simulink model "AirDragTorque"  (R2024b)
settings: Solver=ode8  StartTime=0.0  StopTime=1000  FixedStep=0.1  RelTol=1e-3
undefined symbols (not defined in the file or in its folder): Earth, env, IC, orb, sat
libraries: matrix_library x14
settings Model: Creator=eleon  LastModifiedBy=eleon

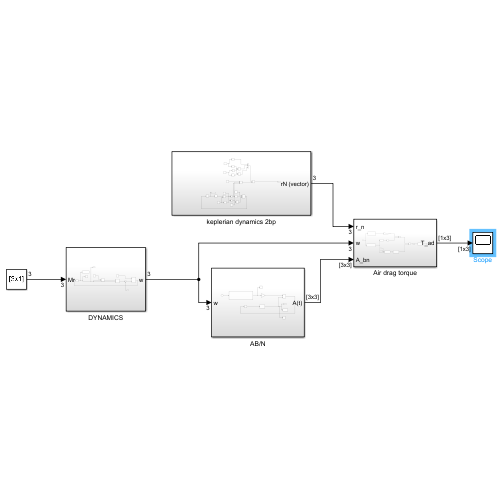
[thumbnail: Simulink's stored preview of the top-level diagram]
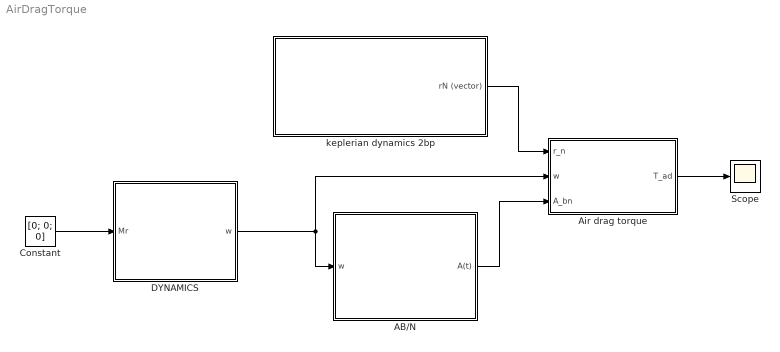
== system AirDragTorque ==
  AB/N : Subsystem
  Air drag torque : Subsystem
  Constant : Constant  Value=[0; 0; 0]
  DYNAMICS : Subsystem
  Scope : Scope
  keplerian dynamics 2bp : Subsystem
  wires:
  Air drag torque/1(T_ad) -> Scope/1
  DYNAMICS/1(w) -> AB/N/1(w), Air drag torque/2(w)
  AB/N/1(A(t)) -> Air drag torque/3(A_bn)
  Constant/1 -> DYNAMICS/1(Mr)
  keplerian dynamics 2bp/1(rN (vector)) -> Air drag torque/1(r_n)

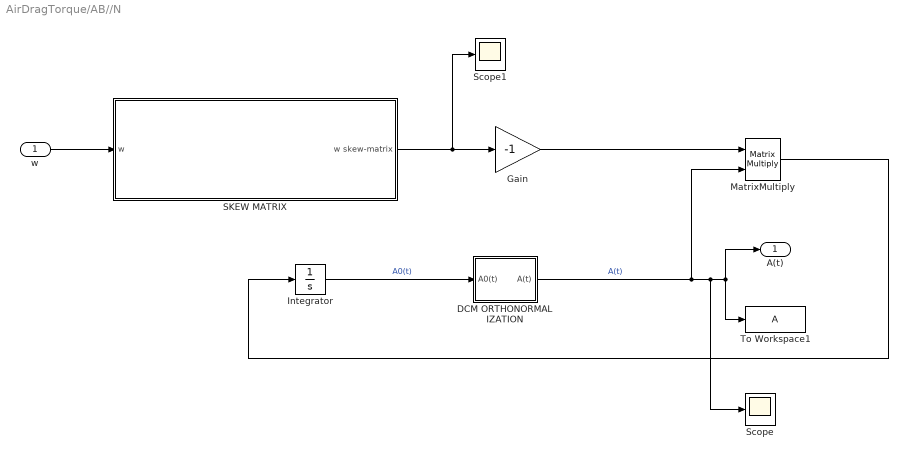
== system AirDragTorque/AB//N ==
  w : Inport
  DCM ORTHONORMALIZATION : Subsystem
  Gain : Gain  Gain=-1
  Integrator : Integrator  InitialCondition=eye(3)
  MatrixMultiply : Product  Multiplication=Matrix(*)
  SKEW MATRIX : Subsystem
  Scope : Scope
  Scope1 : Scope
  To Workspace1 : ToWorkspace  VariableName=A  SampleTime=-1
  A(t) : Outport
  wires:
  w/1 -> SKEW MATRIX/1(w)
  Gain/1 -> MatrixMultiply/1
  MatrixMultiply/1 -> Integrator/1
  SKEW MATRIX/1(w skew-matrix) -> Scope1/1, Gain/1
  Integrator/1 -> DCM ORTHONORMALIZATION/1(A0(t))  "A0(t)"
  DCM ORTHONORMALIZATION/1(A(t)) -> Scope/1, A(t)/1, To Workspace1/1, MatrixMultiply/2  "A(t)"

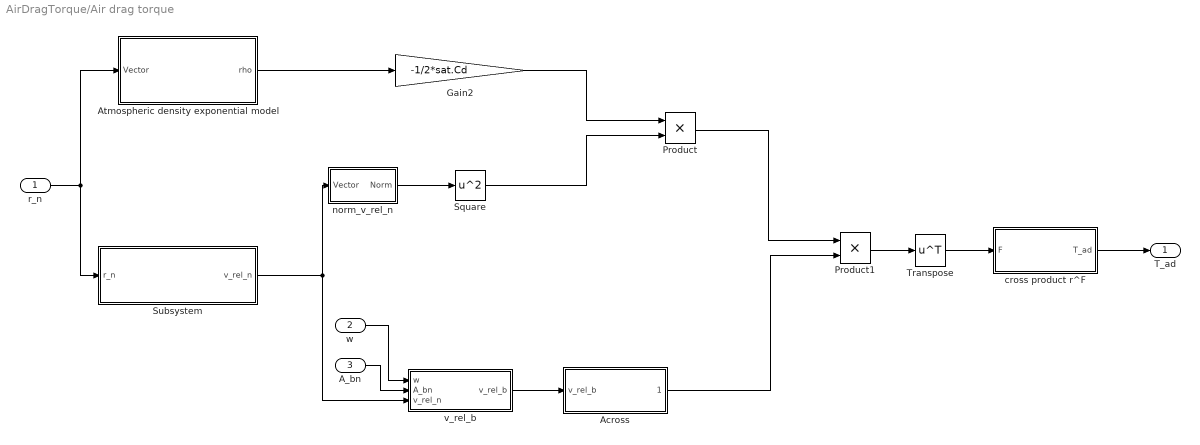
== system AirDragTorque/Air drag torque ==
  r_n : Inport
  w : Inport  Port=2
  A_bn : Inport  Port=3
  Across : Subsystem
  Atmospheric density exponential model : Subsystem
  Gain2 : Gain  Gain=-1/2*sat.Cd
  Product : Product
  Product1 : Product
  Square : Math  Operator=square
  Subsystem : Subsystem
  Transpose : Math  Operator=transpose
  cross product r^F : Subsystem
  norm_v_rel_n : Subsystem
  v_rel_b : Subsystem
  T_ad : Outport
  wires:
  r_n/1 -> Subsystem/1(r_n), Atmospheric density exponential model/1(Vector)
  Atmospheric density exponential model/1(rho) -> Gain2/1
  norm_v_rel_n/1(Norm) -> Square/1
  w/1 -> v_rel_b/1(w)
  A_bn/1 -> v_rel_b/2(A_bn)
  v_rel_b/1(v_rel_b) -> Across/1(v_rel_b)
  cross product r^F/1(T_ad) -> T_ad/1
  Gain2/1 -> Product/1
  Square/1 -> Product/2
  Product/1 -> Product1/1
  Across/1(" ") -> Product1/2
  Product1/1 -> Transpose/1
  Transpose/1 -> cross product r^F/1(F)
  Subsystem/1(v_rel_n) -> norm_v_rel_n/1(Vector), v_rel_b/3(v_rel_n)

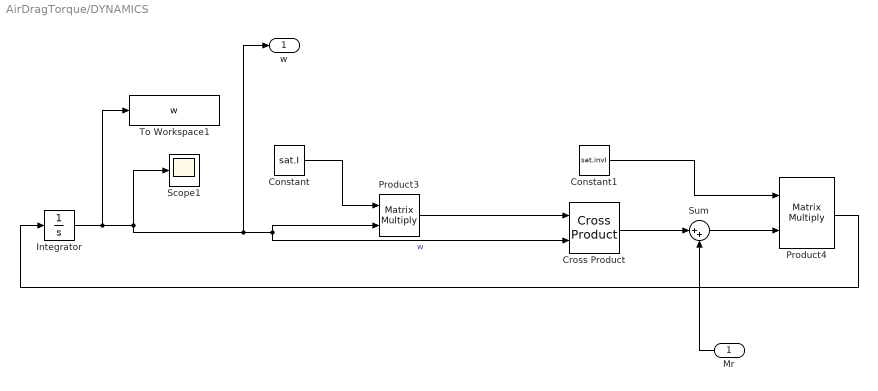
== system AirDragTorque/DYNAMICS ==
  Mr : Inport
  Constant : Constant  Value=sat.I
  Constant1 : Constant  Value=sat.invI
  Cross Product : matrix_library/Cross Product
  Integrator : Integrator  InitialCondition=IC.w0
  Product3 : Product  Multiplication=Matrix(*)
  Product4 : Product  Multiplication=Matrix(*)
  Scope1 : Scope
  Sum : Sum  Inputs=|++
  To Workspace1 : ToWorkspace  VariableName=w  SampleTime=-1
  w : Outport
  wires:
  Sum/1 -> Product4/2
  Cross Product/1 -> Sum/1
  Mr/1 -> Sum/2
  Product4/1 -> Integrator/1
  Product3/1 -> Cross Product/1
  Constant/1 -> Product3/1
  Integrator/1 -> To Workspace1/1, w/1, Product3/2, Cross Product/2, Scope1/1  "w"
  Constant1/1 -> Product4/1

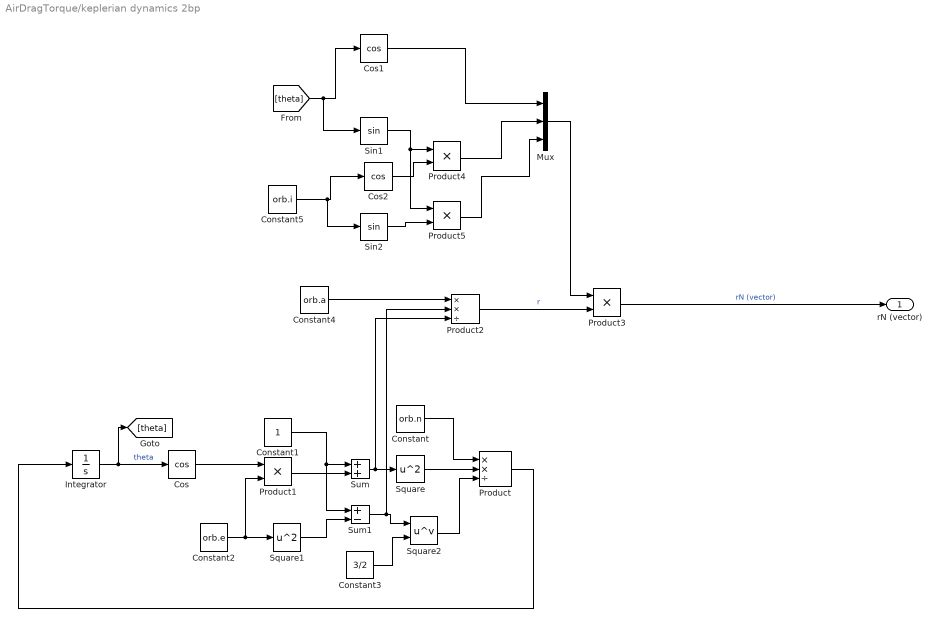
== system AirDragTorque/keplerian dynamics 2bp ==
  Constant : Constant  Value=orb.n
  Constant1 : Constant
  Constant2 : Constant  Value=orb.e
  Constant3 : Constant  Value=3/2
  Constant4 : Constant  Value=orb.a
  Constant5 : Constant  Value=orb.i
  Cos : Trigonometry  Operator=cos
  Cos1 : Trigonometry  Operator=cos
  Cos2 : Trigonometry  Operator=cos
  Integrator : Integrator  InitialCondition=IC.theta
  Mux : Mux  Inputs=3
  Product : Product  Inputs=**/
  Product{1,3..5} (4 alike) : Product
  Product2 : Product  Inputs=**/
  Sin1 : Trigonometry
  Sin2 : Trigonometry
  Square : Math  Operator=square
  Square1 : Math  Operator=square
  Square2 : Math  Operator=pow
  Sum : Sum  Inputs=+|+
  Sum1 : Sum  Inputs=+|-
  rN (vector) : Outport
  wires:
  Constant2/1 -> Square1/1, Product1/2
  Cos2/1 -> Product4/2
  Sum1/1 -> Product2/2, Square2/1
  [theta] -> Sin1/1, Cos1/1
  Product1/1 -> Sum/2
  Constant1/1 -> Sum1/1, Sum/1
  Product5/1 -> Mux/3
  Product/1 -> Integrator/1
  Mux/1 -> Product3/1
  Integrator/1 -> [theta], Cos/1  "theta"
  Sin1/1 -> Product4/1, Product5/1
  Sum/1 -> Product2/3, Square/1
  Square/1 -> Product/2
  Constant4/1 -> Product2/1
  Product2/1 -> Product3/2  "r"
  Constant3/1 -> Square2/2
  Cos1/1 -> Mux/1
  Product3/1 -> rN (vector)/1  "rN (vector)"
  Square1/1 -> Sum1/2
  Square2/1 -> Product/3
  Cos/1 -> Product1/1
  Constant5/1 -> Sin2/1, Cos2/1
  Sin2/1 -> Product5/2
  Constant/1 -> Product/1
  Product4/1 -> Mux/2

== system AirDragTorque/AB//N/DCM ORTHONORMALIZATION ==
  A0(t) : Inport
  Gain : Gain  Gain=3/2
  Gain1 : Gain  Gain=-1/2
  Matrix Multiply : Product  Inputs=3  Multiplication=Matrix(*)
  Sum : Sum  Inputs=|++
  Transpose : Math  Operator=transpose
  A(t) : Outport
  wires:
  A0(t)/1 -> Matrix Multiply/3, Transpose/1, Matrix Multiply/1, Gain/1
  Transpose/1 -> Matrix Multiply/2
  Gain/1 -> Sum/1
  Matrix Multiply/1 -> Gain1/1
  Sum/1 -> A(t)/1
  Gain1/1 -> Sum/2

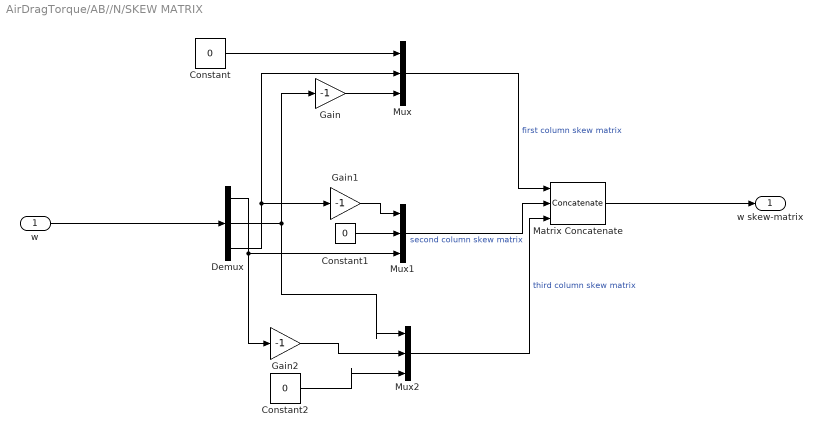
== system AirDragTorque/AB//N/SKEW MATRIX ==
  w : Inport
  Constant : Constant  Value=0
  Constant1 : Constant  Value=0
  Constant2 : Constant  Value=0
  Demux : Demux  Outputs=3
  Gain : Gain  Gain=-1
  Gain1 : Gain  Gain=-1
  Gain2 : Gain  Gain=-1
  Matrix Concatenate : Concatenate  NumInputs=3  Mode=Multidimensional array  ConcatenateDimension=2
  Mux : Mux  Inputs=3
  Mux1 : Mux  Inputs=3
  Mux2 : Mux  Inputs=3
  w skew-matrix : Outport
  wires:
  w/1 -> Demux/1
  Matrix Concatenate/1 -> w skew-matrix/1
  Constant/1 -> Mux/1
  Gain/1 -> Mux/3
  Demux/3 -> Gain1/1, Mux/2
  Demux/2 -> Mux2/1, Gain/1
  Mux/1 -> Matrix Concatenate/1  "first column skew matrix"
  Constant1/1 -> Mux1/2
  Gain1/1 -> Mux1/1
  Demux/1 -> Gain2/1, Mux1/3
  Mux1/1 -> Matrix Concatenate/2  "second column skew matrix"
  Gain2/1 -> Mux2/2
  Constant2/1 -> Mux2/3
  Mux2/1 -> Matrix Concatenate/3  "third column skew matrix"

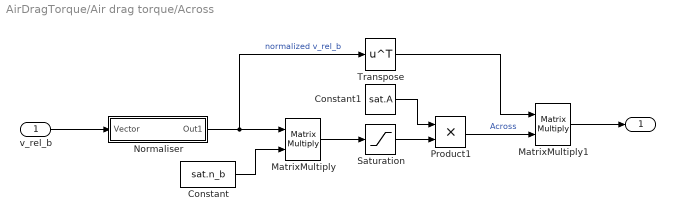
== system AirDragTorque/Air drag torque/Across ==
  v_rel_b : Inport
  Constant : Constant  Value=sat.n_b
  Constant1 : Constant  Value=sat.A
  MatrixMultiply : Product  Multiplication=Matrix(*)
  MatrixMultiply1 : Product  Multiplication=Matrix(*)
  Normaliser : Subsystem
  Product1 : Product
  Saturation : Saturate  UpperLimit=1  LowerLimit=0
  Transpose : Math  Operator=transpose
  " " : Outport
  wires:
  v_rel_b/1 -> Normaliser/1(Vector)
  Constant/1 -> MatrixMultiply/2
  Normaliser/1(Out1) -> Transpose/1, MatrixMultiply/1  "normalized v_rel_b"
  MatrixMultiply/1 -> Saturation/1
  Saturation/1 -> Product1/2
  Constant1/1 -> Product1/1
  Product1/1 -> MatrixMultiply1/2  "Across"
  MatrixMultiply1/1 -> " "/1
  Transpose/1 -> MatrixMultiply1/1

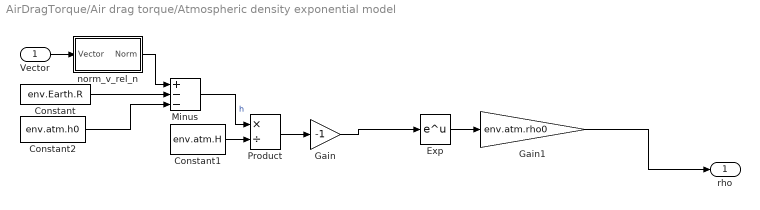
== system AirDragTorque/Air drag torque/Atmospheric density exponential model ==
  Vector : Inport
  Constant : Constant  Value=env.Earth.R
  Constant1 : Constant  Value=env.atm.H
  Constant2 : Constant  Value=env.atm.h0
  Exp : Math
  Gain : Gain  Gain=-1
  Gain1 : Gain  Gain=env.atm.rho0
  Minus : Sum  Inputs=+--
  Product : Product  Inputs=*/
  norm_v_rel_n : Subsystem
  rho : Outport
  wires:
  Constant/1 -> Minus/2
  Gain/1 -> Exp/1
  Exp/1 -> Gain1/1
  Constant1/1 -> Product/2
  Minus/1 -> Product/1  "h"
  Product/1 -> Gain/1
  Gain1/1 -> rho/1
  Vector/1 -> norm_v_rel_n/1(Vector)
  Constant2/1 -> Minus/3
  norm_v_rel_n/1(Norm) -> Minus/1

== system AirDragTorque/Air drag torque/Subsystem ==
  r_n : Inport
  Constant : Constant  Value=[0, 0, env. Earth.omega]
  Cross Product : matrix_library/Cross Product
  Derivative : Derivative
  Minus : Sum  Inputs=+-
  v_rel_n : Outport
  wires:
  Derivative/1 -> Minus/1  "V_s/c_n"
  Constant/1 -> Cross Product/1
  Cross Product/1 -> Minus/2  "V_atm_n"
  Minus/1 -> v_rel_n/1  "v_rel_n"
  r_n/1 -> Derivative/1, Cross Product/2

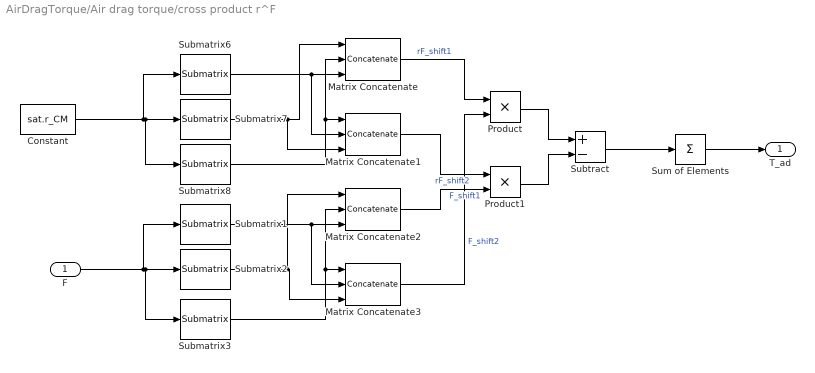
== system AirDragTorque/Air drag torque/cross product r^F ==
  F : Inport
  Constant : Constant  Value=sat.r_CM
  Matrix Concatenate{,1..3} (4 alike) : Concatenate  NumInputs=3  Mode=Multidimensional array  ConcatenateDimension=2
  Product : Product
  Product1 : Product
  Submatrix1 : matrix_library/Submatrix  RowSpan=All rows  RowStartMode=Index  RowStartIndex=1  RowEndMode=Last  RowEndIndex=1  ColSpan=One column  ColStartMode=Index  ColStartIndex=1  ColEndMode=Last  ColEndIndex=1
  Submatrix2 : matrix_library/Submatrix  RowSpan=All rows  RowStartMode=First  RowStartIndex=1  RowEndMode=Last  RowEndIndex=1  ColSpan=One column  ColStartMode=Index  ColStartIndex=2  ColEndMode=Last  ColEndIndex=1
  Submatrix3 : matrix_library/Submatrix  RowSpan=All rows  RowStartMode=Index  RowStartIndex=3  RowEndMode=Last  RowEndIndex=1  ColSpan=One column  ColStartMode=Index  ColStartIndex=3  ColEndMode=Last  ColEndIndex=1
  Submatrix6 : matrix_library/Submatrix  RowSpan=All rows  RowStartMode=Index  RowStartIndex=1  RowEndMode=Last  RowEndIndex=1  ColSpan=One column  ColStartMode=Index  ColStartIndex=1  ColEndMode=Last  ColEndIndex=1
  Submatrix7 : matrix_library/Submatrix  RowSpan=All rows  RowStartMode=First  RowStartIndex=1  RowEndMode=Last  RowEndIndex=1  ColSpan=One column  ColStartMode=Index  ColStartIndex=2  ColEndMode=Last  ColEndIndex=1
  Submatrix8 : matrix_library/Submatrix  RowSpan=All rows  RowStartMode=Index  RowStartIndex=3  RowEndMode=Last  RowEndIndex=1  ColSpan=One column  ColStartMode=Index  ColStartIndex=3  ColEndMode=Last  ColEndIndex=1
  Subtract : Sum  Inputs=+-
  Sum of Elements : Sum  Inputs=+  CollapseMode=Specified dimension
  T_ad : Outport
  wires:
  Submatrix7/1 -> Matrix Concatenate/1, Matrix Concatenate1/3
  Submatrix6/1 -> Matrix Concatenate1/2, Matrix Concatenate/3
  Submatrix8/1 -> Matrix Concatenate1/1, Matrix Concatenate/2
  Constant/1 -> Submatrix7/1, Submatrix8/1, Submatrix6/1
  Matrix Concatenate/1 -> Product/1  "rF_shift1"
  Matrix Concatenate1/1 -> Product1/1  "rF_shift2"
  Submatrix3/1 -> Matrix Concatenate3/1, Matrix Concatenate2/2
  Submatrix2/1 -> Matrix Concatenate3/3, Matrix Concatenate2/1
  F/1 -> Submatrix2/1, Submatrix3/1, Submatrix1/1
  Submatrix1/1 -> Matrix Concatenate3/2, Matrix Concatenate2/3
  Matrix Concatenate2/1 -> Product1/2  "F_shift1"
  Matrix Concatenate3/1 -> Product/2  "F_shift2"
  Product/1 -> Subtract/1
  Product1/1 -> Subtract/2
  Subtract/1 -> Sum of Elements/1
  Sum of Elements/1 -> T_ad/1

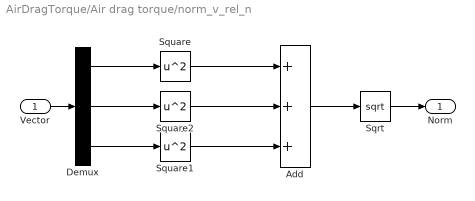
== system AirDragTorque/Air drag torque/norm_v_rel_n ==
  Vector : Inport
  Add : Sum  Inputs=+++
  Demux : Demux  Outputs=3
  Sqrt : Sqrt
  Square : Math  Operator=square
  Square1 : Math  Operator=square
  Square2 : Math  Operator=square
  Norm : Outport
  wires:
  Square/1 -> Add/1
  Add/1 -> Sqrt/1
  Demux/3 -> Square1/1
  Square2/1 -> Add/2
  Square1/1 -> Add/3
  Demux/1 -> Square/1
  Demux/2 -> Square2/1
  Vector/1 -> Demux/1
  Sqrt/1 -> Norm/1

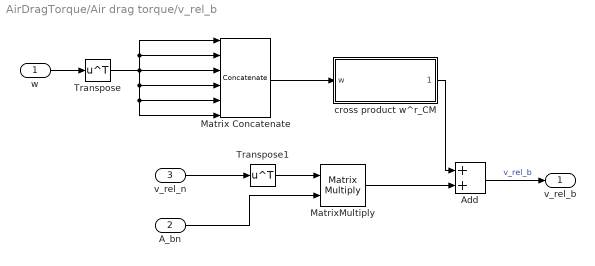
== system AirDragTorque/Air drag torque/v_rel_b ==
  w : Inport
  A_bn : Inport  Port=2
  v_rel_n : Inport  Port=3
  Add : Sum
  Matrix Concatenate : Concatenate  NumInputs=6  Mode=Multidimensional array
  MatrixMultiply : Product  Multiplication=Matrix(*)
  Transpose : Math  Operator=transpose
  Transpose1 : Math  Operator=transpose
  cross product w^r_CM : Subsystem
  v_rel_b : Outport
  wires:
  A_bn/1 -> MatrixMultiply/2
  v_rel_n/1 -> Transpose1/1
  MatrixMultiply/1 -> Add/2
  w/1 -> Transpose/1
  Add/1 -> v_rel_b/1  "v_rel_b"
  cross product w^r_CM/1(" ") -> Add/1
  Transpose/1 -> Matrix Concatenate/6, Matrix Concatenate/5, Matrix Concatenate/4, Matrix Concatenate/2, Matrix Concatenate/1, Matrix Concatenate/3
  Matrix Concatenate/1 -> cross product w^r_CM/1(w)
  Transpose1/1 -> MatrixMultiply/1

== system AirDragTorque/Air drag torque/Across/Normaliser ==
  Vector : Inport
  Constant : Constant  Value=[0; 0; 0]
  Norm1 : Subsystem
  Protected Division : Subsystem
  Switch : Switch  Criteria=u2 ~= 0  SaturateOnIntegerOverflow=off  InputSameDT=off
  Out1 : Outport
  wires:
  Norm1/1(Norm) -> Switch/2, Protected Division/2(Norm)  "norm_r"
  Switch/1 -> Out1/1
  Protected Division/1(Out1) -> Switch/1
  Vector/1 -> Protected Division/1(Vector), Norm1/1(Vector)
  Constant/1 -> Switch/3

== system AirDragTorque/Air drag torque/Atmospheric density exponential model/norm_v_rel_n ==
  Vector : Inport
  Add : Sum  Inputs=+++
  Demux : Demux  Outputs=3
  Sqrt : Sqrt
  Square : Math  Operator=square
  Square1 : Math  Operator=square
  Square2 : Math  Operator=square
  Norm : Outport
  wires:
  Square/1 -> Add/1
  Add/1 -> Sqrt/1
  Demux/3 -> Square1/1
  Square2/1 -> Add/2
  Square1/1 -> Add/3
  Demux/1 -> Square/1
  Demux/2 -> Square2/1
  Vector/1 -> Demux/1
  Sqrt/1 -> Norm/1

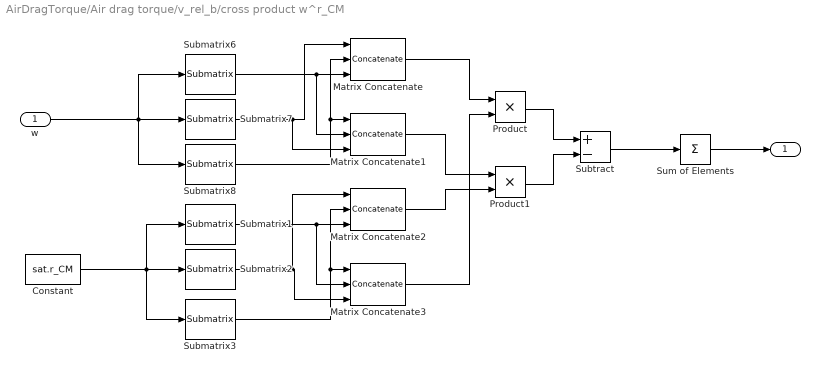
== system AirDragTorque/Air drag torque/v_rel_b/cross product w^r_CM ==
  w : Inport
  Constant : Constant  Value=sat.r_CM
  Matrix Concatenate{,1..3} (4 alike) : Concatenate  NumInputs=3  Mode=Multidimensional array  ConcatenateDimension=2
  Product : Product
  Product1 : Product
  Submatrix1 : matrix_library/Submatrix  RowSpan=All rows  RowStartMode=Index  RowStartIndex=1  RowEndMode=Last  RowEndIndex=1  ColSpan=One column  ColStartMode=Index  ColStartIndex=1  ColEndMode=Last  ColEndIndex=1
  Submatrix2 : matrix_library/Submatrix  RowSpan=All rows  RowStartMode=First  RowStartIndex=1  RowEndMode=Last  RowEndIndex=1  ColSpan=One column  ColStartMode=Index  ColStartIndex=2  ColEndMode=Last  ColEndIndex=1
  Submatrix3 : matrix_library/Submatrix  RowSpan=All rows  RowStartMode=Index  RowStartIndex=3  RowEndMode=Last  RowEndIndex=1  ColSpan=One column  ColStartMode=Index  ColStartIndex=3  ColEndMode=Last  ColEndIndex=1
  Submatrix6 : matrix_library/Submatrix  RowSpan=All rows  RowStartMode=Index  RowStartIndex=1  RowEndMode=Last  RowEndIndex=1  ColSpan=One column  ColStartMode=Index  ColStartIndex=1  ColEndMode=Last  ColEndIndex=1
  Submatrix7 : matrix_library/Submatrix  RowSpan=All rows  RowStartMode=First  RowStartIndex=1  RowEndMode=Last  RowEndIndex=1  ColSpan=One column  ColStartMode=Index  ColStartIndex=2  ColEndMode=Last  ColEndIndex=1
  Submatrix8 : matrix_library/Submatrix  RowSpan=All rows  RowStartMode=Index  RowStartIndex=3  RowEndMode=Last  RowEndIndex=1  ColSpan=One column  ColStartMode=Index  ColStartIndex=3  ColEndMode=Last  ColEndIndex=1
  Subtract : Sum  Inputs=+-
  Sum of Elements : Sum  Inputs=+  CollapseMode=Specified dimension
  " " : Outport
  wires:
  Submatrix7/1 -> Matrix Concatenate/1, Matrix Concatenate1/3
  Submatrix6/1 -> Matrix Concatenate1/2, Matrix Concatenate/3
  Submatrix8/1 -> Matrix Concatenate1/1, Matrix Concatenate/2
  Constant/1 -> Submatrix3/1, Submatrix2/1, Submatrix1/1
  Matrix Concatenate/1 -> Product/1
  Matrix Concatenate1/1 -> Product1/1
  Submatrix3/1 -> Matrix Concatenate3/1, Matrix Concatenate2/2
  Submatrix2/1 -> Matrix Concatenate3/3, Matrix Concatenate2/1
  w/1 -> Submatrix6/1, Submatrix8/1, Submatrix7/1
  Submatrix1/1 -> Matrix Concatenate3/2, Matrix Concatenate2/3
  Matrix Concatenate2/1 -> Product1/2
  Matrix Concatenate3/1 -> Product/2
  Product/1 -> Subtract/1
  Product1/1 -> Subtract/2
  Subtract/1 -> Sum of Elements/1
  Sum of Elements/1 -> " "/1

== system AirDragTorque/Air drag torque/Across/Normaliser/Norm1 ==
  Vector : Inport
  Add : Sum  Inputs=+++
  Demux : Demux  Outputs=3
  Sqrt : Sqrt
  Square : Math  Operator=square
  Square1 : Math  Operator=square
  Square2 : Math  Operator=square
  Norm : Outport
  wires:
  Square/1 -> Add/1
  Add/1 -> Sqrt/1
  Demux/3 -> Square1/1
  Square2/1 -> Add/2
  Square1/1 -> Add/3
  Demux/1 -> Square/1
  Demux/2 -> Square2/1
  Vector/1 -> Demux/1
  Sqrt/1 -> Norm/1

== system AirDragTorque/Air drag torque/Across/Normaliser/Protected Division ==
  Vector : Inport
  Norm : Inport  Port=2
  Constant : Constant  Value=eps
  Divide : Product  Inputs=*/
  Switch : Switch  Criteria=u2 ~= 0  SaturateOnIntegerOverflow=off  InputSameDT=off
  Out1 : Outport
  wires:
  Divide/1 -> Out1/1
  Vector/1 -> Divide/1
  Norm/1 -> Switch/1, Switch/2
  Switch/1 -> Divide/2
  Constant/1 -> Switch/3
